simulink model "carmodel"  (R2021b)
settings: Solver=VariableStepAuto  StartTime=0.0  StopTime=100  RelTol=1e-3
libraries: fuzblock x1
settings Model: Creator=radov  LastModifiedBy=radov

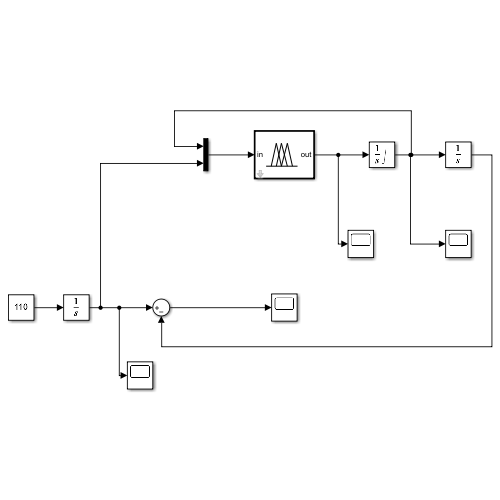
[thumbnail: Simulink's stored preview of the top-level diagram]
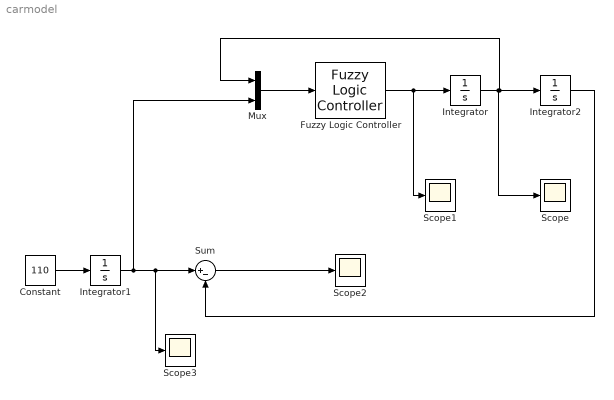
== system carmodel ==
  Constant : Constant  Value=110
  Fuzzy Logic Controller : fuzblock/Fuzzy Logic  Controller  FIS=car  OutputSampleNumber=101  DataType=double  FuzzifiedInputs=off  RuleFiringStrengths=off  RuleOutputs=off  AggregatedOutputs=off  SimulateUsing=Interpreted execution  OutOfRangeInputValueMessage=warning  NoRuleFiredMessage=warning  EmptyOutputFuzzySetMessage=warning
  Integrator : Integrator  LimitOutput=on  UpperSaturationLimit=180  LowerSaturationLimit=0
  Integrator1 : Integrator
  Integrator2 : Integrator
  Mux : Mux  Inputs=2
  Scope{,1..3} (4 alike) : Scope
  Sum : Sum  Inputs=|+-
  wires:
  Mux/1 -> Fuzzy Logic Controller/1
  Fuzzy Logic Controller/1 -> Scope1/1, Integrator/1
  Integrator/1 -> Integrator2/1, Mux/1, Scope/1
  Constant/1 -> Integrator1/1
  Integrator1/1 -> Mux/2, Scope3/1, Sum/1
  Integrator2/1 -> Sum/2
  Sum/1 -> Scope2/1
